simulink model "PV_SolarCell"  (R2019a)
settings: Solver=VariableStepAuto  StartTime=0.0  StopTime=10.0  RelTol=1e-3
libraries: fl_lib x5, nesl_utility x4, simulink x3, ee_lib x1
settings Model: Creator=Lenovo  LastModifiedBy=Lenovo

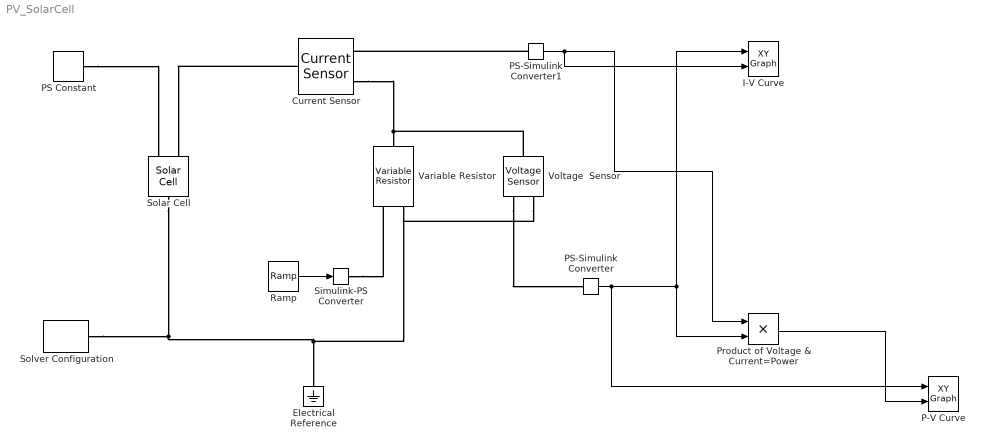
== system PV_SolarCell ==
  "Current Sensor " : fl_lib/Electrical/Electrical Sensors/Current Sensor
  Electrical Reference : fl_lib/Electrical/Electrical Elements/Electrical Reference
  I-V Curve : simulink/Sinks/XY Graph  xmin=0  xmax=0.7  ymin=0  ymax=8  st=-1
  P-V Curve : simulink/Sinks/XY Graph  xmin=0  xmax=0.7  ymin=0  ymax=4  st=-1
  "PS Constant " : fl_lib/Physical Signals/Sources/PS Constant  constant=1000
  PS-Simulink Converter : nesl_utility/PS-Simulink Converter  PhysicalDomain=network_engine_domain  SubClassName=ps_output  LeftPortType=input  RightPortType=output  PseudoPeriodic=off  Frequencies=[]  Unit=1  AffineConversion=off
  PS-Simulink Converter1 : nesl_utility/PS-Simulink Converter  PhysicalDomain=network_engine_domain  SubClassName=ps_output  LeftPortType=input  RightPortType=output  PseudoPeriodic=off  Frequencies=[]  Unit=1  AffineConversion=off
  Product of Voltage & Current=Power : Product
  "Ramp " : simulink/Sources/Ramp  slope=1  start=0  InitialOutput=0
  Simulink-PS Converter : nesl_utility/Simulink-PS Converter  PhysicalDomain=network_engine_domain  SubClassName=ps_input  LeftPortType=input  RightPortType=output  PseudoPeriodic=off  Frequencies=[]  NoiseDistribution=none  NoiseParameters=[]  Unit=1  AffineConversion=off  FilteringAndDerivatives=provide  SimscapeFilterOrder=1  InputFilterTimeConstant=0.001  UdotUserProvided=0
  Solar Cell : ee_lib/Sources/Solar Cell  prm=1  Isc=7.34 A  Voc=0.6 V  Is=1e-6 A  Is2=0 A  Iph=7.34 A  Ir0=1000 W/m^2  ec=1.5  N2=2  Rs=0 Ohm  Rp=inf Ohm  N_series=1  TIPH1=0 1/K  EG=1.11 eV  TXIS1=3  TXIS2=3  TRS1=0  TRP1=0  Tmeas=25 degC  TFIXED=25 degC  thermal_mass=100 J/K  initial_temperature=25 degC
      settings: SourceProductName=Simscape Electrical  SourceProductBaseCode=PS
  "Solver Configuration " : nesl_utility/Solver Configuration  PhysicalDomain=network_engine_domain  SubClassName=solver  LeftPortType=input  RightPortType=generic  Tones=[]  Harmonics=[]  SimulateNoise=off  Profile=off  UseLocalSampling=off  EnableSwitchedLinearOptims=on  FrequencyDomain=off  UseCCode=off  RelTol=0.001  AbsTol=1e-06  MinStep=1e-09  ToWorkspace=off  RevertToSquareIcSolve=off  NumHomotopyIterations=100  PhasorMode=off  PhasorModeNumHarmonics=1  DoDC=off  ResidualTolerance=1e-09  UseLocalSolver=off  LocalSolverChoice=NE_BACKWARD_EULER_ADVANCER  LocalSolverSampleTime=0.001  DoFixedCost=off  MaxNonlinIter=3  MaxModeIter=2  LinearAlgebra=auto  EquationFormulation=NE_TIME_EF  DelaysMemoryBudget=1024  AutomaticFiltering=on  FilteringTimeConstant=0.001  PartitionStorageMethod=AS_NEEDED  PartitionMemoryBudget=1024  PartitionMethod=ROBUST
  "Variable Resistor " : fl_lib/Electrical/Electrical Elements/Variable Resistor  Rmin=0 Ohm  i_specify=off  i_priority=None  i=0 A  i_nominal_specify=off  i_nominal_unit=A  i_nominal_value=1  v_specify=off  v_priority=None  v=0 V  v_nominal_specify=off  v_nominal_unit=V  v_nominal_value=1
  Voltage  Sensor : fl_lib/Electrical/Electrical Sensors/Voltage Sensor
  wires:
  "Ramp "/1 -> Simulink-PS Converter/1
  PS-Simulink Converter1/1 -> I-V Curve/2, Product of Voltage & Current=Power/1
  PS-Simulink Converter/1 -> P-V Curve/1, Product of Voltage & Current=Power/2, I-V Curve/1
  Product of Voltage & Current=Power/1 -> P-V Curve/2
  connections:
  "PS Constant "/RConn1 -- Solar Cell/LConn1
  "Current Sensor "/LConn1 -- Solar Cell/LConn2
  Simulink-PS Converter/RConn1 -- "Variable Resistor "/LConn1
  Solar Cell/RConn1 -- "Solver Configuration "/RConn1 -- Voltage  Sensor/RConn2 -- "Variable Resistor "/LConn2 -- Electrical Reference/LConn1
  "Current Sensor "/RConn2 -- Voltage  Sensor/LConn1 -- "Variable Resistor "/RConn1
  PS-Simulink Converter1/LConn1 -- "Current Sensor "/RConn1
  Voltage  Sensor/RConn1 -- PS-Simulink Converter/LConn1
